simulink model "NonLinearSystems_Project_Control"  (R2022a)
settings: Solver=ode45  StartTime=0.0  StopTime=30  RelTol=1e-6
settings Model: Creator=User  LastModifiedBy=User
settings SolverCC: MaxConsecutiveMinStep=3

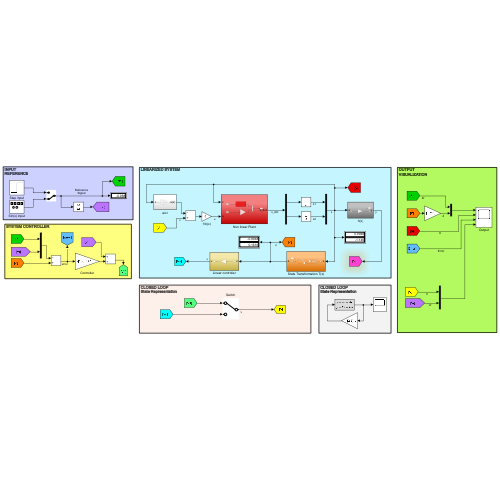
[thumbnail: Simulink's stored preview of the top-level diagram]
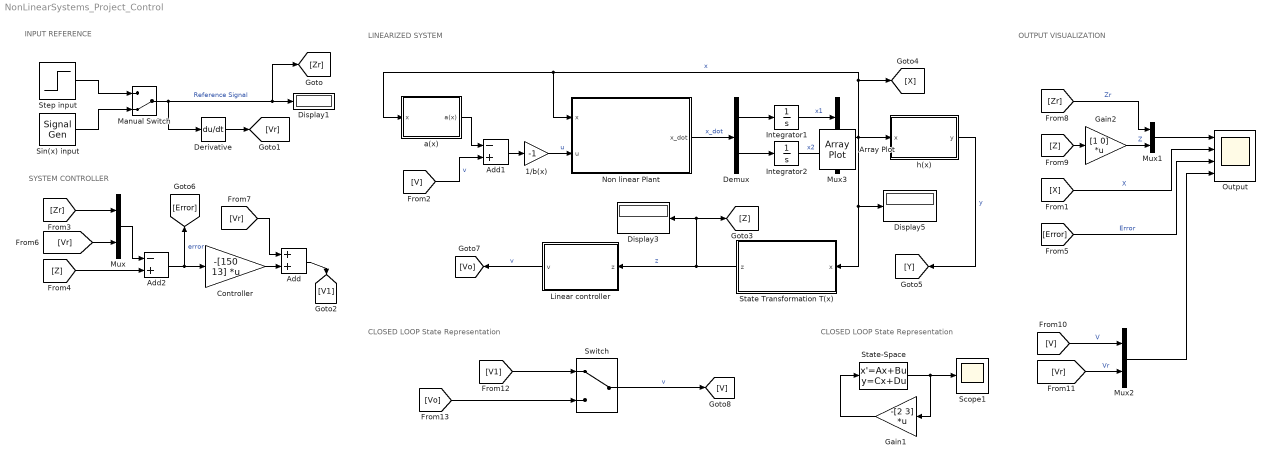
== system NonLinearSystems_Project_Control ==
  note: INPUT
      | REFERENCE
  note: LINEARIZED SYSTEM
  note: CLOSED LOOP
      | State Representation
  note: OUTPUT
      | VISUALIZATION
  note: SYSTEM CONTROLLER
  note: CLOSED LOOP
      | State Representation
  1/b(x) : Gain  Gain=-1
  Add : Sum
  Add1 : Sum  Inputs=-+
  Add2 : Sum  Inputs=-+
  Controller : Gain  Gain=-[150 13]  Multiplication=Matrix(K*u)
  Demux : Demux  Outputs=2
  Derivative : Derivative
  Display1 : Display
  Display3 : Display
  Display5 : Display
  Gain1 : Gain  Gain=-[2 3]  Multiplication=Matrix(K*u)
  Gain2 : Gain  Gain=[1 0]  Multiplication=Matrix(K*u)
  Integrator1 : Integrator  InitialCondition=1
  Integrator2 : Integrator
  Linear controller : Subsystem
  Manual Switch : ManualSwitch  CurrentSetting=0
  Mux{,1..3} (4 alike) : Mux  Inputs=2
  Non linear Plant : Subsystem
  Output : Scope  NumInputPorts=4
  Scope1 : Scope
  Sin(x) input : SignalGenerator  Units=rad/sec
  State Transformation T(x) : Subsystem
  State-Space : StateSpace  A=[0 1;0 0]  B=[0;1]  C=[1 0;0 1]  D=[0;0]  InitialCondition=[1;2]
  Step input : Step  Time=2  After=2  SampleTime=0
  Switch : ManualSwitch
  a(x) : Subsystem
  h(x) : Subsystem
  Array Plot : ArrayPlot  IOType=viewer  WindowPosition=[175.000000,148.000000,800.000000,500.000000,]  IsFloating=on  ScopeFrameLocation=window  ShowLegend=on  DefaultConfigurationName=dsp.scopes.ArrayPlotBlockSpecification
  wires:
  Demux/2 -> Integrator2/1
  State Transformation T(x)/1(z) -> [Z], Display3/1, Linear controller/1(z)  "z"
  Integrator1/1 -> Mux3/1  "x1"
  Demux/1 -> Integrator1/1
  Mux3/1 -> Non linear Plant/1(x), a(x)/1(x), [X], State Transformation T(x)/1(x), Display5/1, h(x)/1(x)  "x"
  Integrator2/1 -> Mux3/2  "x2"
  h(x)/1(y) -> [Y]  "y"
  Non linear Plant/1(x_dot) -> Demux/1  "x_dot"
  Step input/1 -> Manual Switch/1
  Sin(x) input/1 -> Manual Switch/2
  Gain1/1 -> State-Space/1
  State-Space/1 -> Scope1/1, Gain1/1
  [V] -> Add1/2  "v"
  Add1/1 -> 1/b(x)/1
  1/b(x)/1 -> Non linear Plant/2(u)  "u"
  Derivative/1 -> [Vr]
  Mux/1 -> Add2/1
  Add2/1 -> Controller/1, [Error]  "error"
  a(x)/1(a(x)) -> Add1/1
  Manual Switch/1 -> [Zr], Display1/1, Derivative/1  "Reference Signal"
  Controller/1 -> Add/2
  Add/1 -> [V1]
  [Zr] -> Mux/1
  [Z] -> Add2/2
  [Vr] -> Mux/2
  [Vr] -> Add/1
  [Z] -> Gain2/1
  Gain2/1 -> Mux1/2  "Z"
  [Zr] -> Mux1/1  "Zr"
  Mux1/1 -> Output/1
  [X] -> Output/2  "X"
  [Error] -> Output/3  "Error"
  [V] -> Mux2/1  "V"
  [Vr] -> Mux2/2  "Vr"
  Mux2/1 -> Output/4
  Linear controller/1(v) -> [Vo]  "v"
  [V1] -> Switch/1
  [Vo] -> Switch/2
  Switch/1 -> [V]  "v"

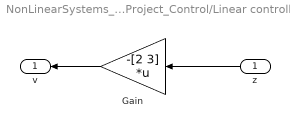
== system NonLinearSystems_Project_Control/Linear controller ==
  z : Inport
  Gain : Gain  Gain=-[2 3]  Multiplication=Matrix(K*u)
  v : Outport
  wires:
  z/1 -> Gain/1
  Gain/1 -> v/1

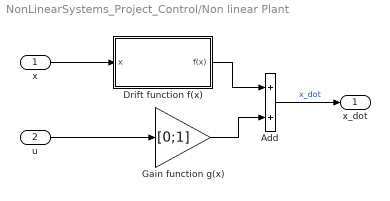
== system NonLinearSystems_Project_Control/Non linear Plant ==
  x : Inport
  u : Inport  Port=2
  Add : Sum
  Drift function f(x) : Subsystem
  Gain function g(x) : Gain  Gain=[0;1]
  x_dot : Outport
  wires:
  Gain function g(x)/1 -> Add/2
  Drift function f(x)/1(f(x)) -> Add/1
  x/1 -> Drift function f(x)/1(x)
  Add/1 -> x_dot/1  "x_dot"
  u/1 -> Gain function g(x)/1

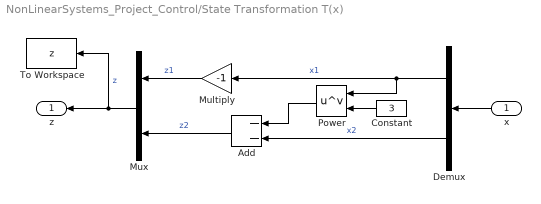
== system NonLinearSystems_Project_Control/State Transformation T(x) ==
  x : Inport
  Add : Sum  Inputs=--
  Constant : Constant  Value=3
  Demux : Demux  Outputs=2
  Multiply : Gain  Gain=-1
  Mux : Mux  Inputs=2
  Power : Math  Operator=pow
  To Workspace : ToWorkspace  VariableName=z  SaveFormat=Timeseries  SampleTime=-1
  z : Outport
  wires:
  Demux/1 -> Power/1, Multiply/1  "x1"
  Multiply/1 -> Mux/1  "z1"
  Constant/1 -> Power/2
  Add/1 -> Mux/2  "z2"
  Power/1 -> Add/1
  Demux/2 -> Add/2  "x2"
  Mux/1 -> To Workspace/1, z/1  "z"
  x/1 -> Demux/1

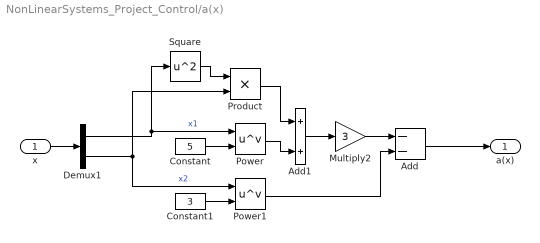
== system NonLinearSystems_Project_Control/a(x) ==
  x : Inport
  Add : Sum  Inputs=--
  Add1 : Sum
  Constant : Constant  Value=5
  Constant1 : Constant  Value=3
  Demux1 : Demux  Outputs=2
  Multiply2 : Gain  Gain=3
  Power : Math  Operator=pow
  Power1 : Math  Operator=pow
  Product : Product
  Square : Math  Operator=square
  a(x) : Outport
  wires:
  Constant/1 -> Power/2
  Demux1/2 -> Power1/1, Product/2  "x2"
  Square/1 -> Product/1
  Demux1/1 -> Square/1, Power/1  "x1"
  Power/1 -> Add1/2
  Add1/1 -> Multiply2/1
  Product/1 -> Add1/1
  x/1 -> Demux1/1
  Constant1/1 -> Power1/2
  Multiply2/1 -> Add/1
  Power1/1 -> Add/2
  Add/1 -> a(x)/1

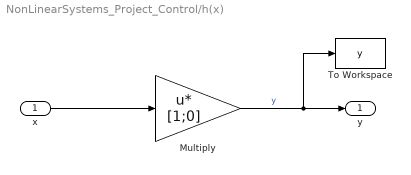
== system NonLinearSystems_Project_Control/h(x) ==
  x : Inport
  Multiply : Gain  Gain=[1;0]  Multiplication=Matrix(u*K)
  To Workspace : ToWorkspace  VariableName=y  SaveFormat=Timeseries  SampleTime=-1
  y : Outport
  wires:
  Multiply/1 -> To Workspace/1, y/1  "y"
  x/1 -> Multiply/1

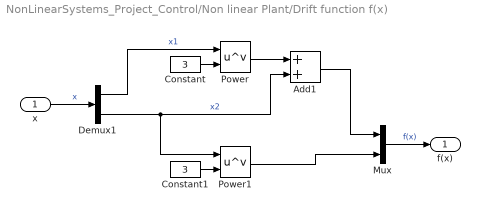
== system NonLinearSystems_Project_Control/Non linear Plant/Drift function f(x) ==
  x : Inport
  Add1 : Sum
  Constant : Constant  Value=3
  Constant1 : Constant  Value=3
  Demux1 : Demux  Outputs=2
  Mux : Mux  Inputs=2
  Power : Math  Operator=pow
  Power1 : Math  Operator=pow
  f(x) : Outport
  wires:
  Constant/1 -> Power/2
  Power/1 -> Add1/1
  Demux1/1 -> Power/1  "x1"
  x/1 -> Demux1/1  "x"
  Add1/1 -> Mux/1
  Constant1/1 -> Power1/2
  Demux1/2 -> Power1/1, Add1/2  "x2"
  Power1/1 -> Mux/2
  Mux/1 -> f(x)/1  "f(x)"
